simulink subsystem "TractionControl"  (R2021b)
settings: Solver=VariableStepAuto  StartTime=0.0  StopTime=10.0  RelTol=1e-3
libraries: simulink x2
settings Model: Creator=tsuyoshi  LastModifiedBy=FEM

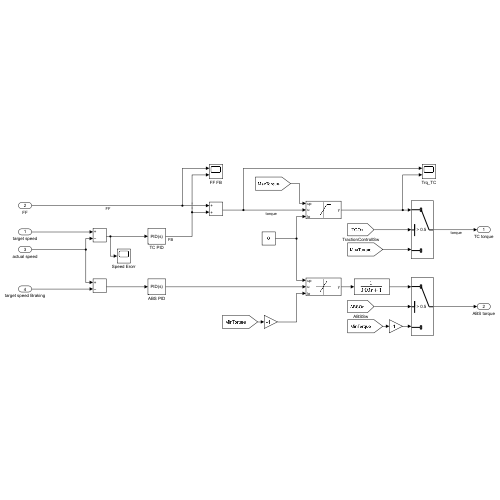
[thumbnail: Simulink's stored preview of the top-level diagram]
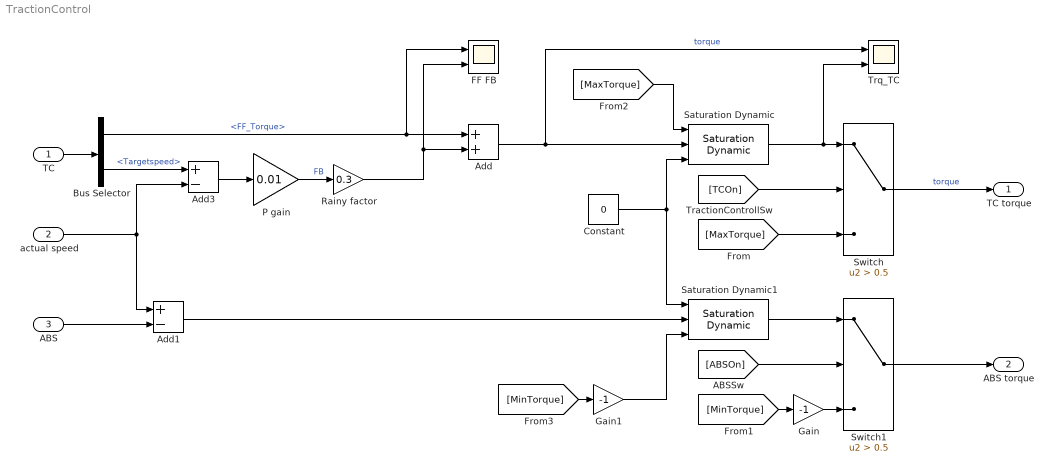
== system TractionControl ==
  TC : Inport
  actual speed : Inport  Port=2
  ABS : Inport  Port=3
  Add : Sum
  Add1 : Sum  Inputs=+-
  Add3 : Sum  Inputs=+-
  Bus Selector : BusSelector  OutputSignals=FF_Torque,Targetspeed
  Constant : Constant  Value=0
  FF FB : Scope  NumInputPorts=2
  Gain : Gain  Gain=-1
  Gain1 : Gain  Gain=-1
  P gain : Gain  Gain=0.01
  Rainy factor : Gain  Gain=0.3
  Saturation Dynamic : simulink/Discontinuities/Saturation Dynamic  OutMin=[]  OutMax=[]  OutDataTypeStr=Inherit: Same as second input  OutDataType=fixdt(1, 16)  OutScaling=2^-10  DoSatur=off
  Saturation Dynamic1 : simulink/Discontinuities/Saturation Dynamic  OutMin=[]  OutMax=[]  OutDataTypeStr=Inherit: Same as second input  OutDataType=fixdt(1, 16)  OutScaling=2^-10  DoSatur=off
  Switch : Switch  Criteria=u2 > Threshold  Threshold=0.5
  Switch1 : Switch  Criteria=u2 > Threshold  Threshold=0.5
  Trq_TC : Scope  NumInputPorts=2
  TC torque : Outport  VectorParamsAs1DForOutWhenUnconnected=off
  ABS torque : Outport  Port=2  VectorParamsAs1DForOutWhenUnconnected=off
  wires:
  Bus Selector/2 -> Add3/1  "<Targetspeed>"
  Saturation Dynamic1/1 -> Switch1/1
  Gain1/1 -> Saturation Dynamic1/3
  [MinTorque] -> Gain1/1
  Add1/1 -> Saturation Dynamic1/2
  Constant/1 -> Saturation Dynamic1/1, Saturation Dynamic/3
  [MaxTorque] -> Saturation Dynamic/1
  [MinTorque] -> Gain/1
  Switch1/1 -> ABS torque/1
  [ABSOn] -> Switch1/2
  Gain/1 -> Switch1/3
  [MaxTorque] -> Switch/3
  [TCOn] -> Switch/2
  ABS/1 -> Add1/2
  Add3/1 -> P gain/1
  TC/1 -> Bus Selector/1
  actual speed/1 -> Add3/2, Add1/1
  Add/1 -> Saturation Dynamic/2, Trq_TC/1  "torque"
  Switch/1 -> TC torque/1  "torque"
  P gain/1 -> Rainy factor/1  "FB"
  Saturation Dynamic/1 -> Switch/1, Trq_TC/2
  Bus Selector/1 -> FF FB/1, Add/1  "<FF_Torque>"
  Rainy factor/1 -> Add/2, FF FB/2
